simulink model "arduino_encoder"  (R2023b)
settings: Solver=FixedStepAuto  StartTime=0.0  StopTime=inf  RelTol=1e-3  EnableMultiTasking=on
undefined symbols (not defined in the file): DiscIntNeverNeededParam
libraries: arduinosensorlib x2
settings Model: ExtModeTrigDuration=2  Creator=yoany  LastModifiedBy=yoany
settings SolverCC: AutoInsertRateTranBlk=on
settings OptimizationCC: EnhancedBackFolding=on  PassReuseOutputArgsAs=Individual arguments  ZeroExternalMemoryAtStartup=off  ZeroInternalMemoryAtStartup=off  MaxStackSize=64  OptimizeBlockOrder=speed  DifferentSizesBufferReuse=on  OptimizationCustomize=off  EfficientTunableParamExpr=on
settings DebuggingCC: ParameterTunabilityLossMsg=error
settings HardwareCC: ProdBitPerPointer=32  ProdBitPerSizeT=32  ProdBitPerPtrDiffT=32  ProdLargestAtomicInteger=Long  ProdLargestAtomicFloat=Double  ProdWordSize=32  ProdHWDeviceType=ARM Compatible->ARM Cortex  UseEmbeddedCoderFeatures=off
settings SFSimCC: MATLABDynamicMemAlloc=off
settings RTWCC: Description=Embedded Coder  SystemTargetFile=ert.tlc  HardwareBoard=Arduino Nano 33 IoT  TemplateMakefile=ert_default_tmf  Toolchain=Arduino ARM  BuildConfiguration=Faster Runs
settings CodeAppCC: ForceParamTrailComments=on  IgnoreCustomStorageClasses=off  OperatorAnnotations=on  SimulinkDataObjDesc=on  SFDataObjDesc=on  InsertBlockDesc=on
settings ERTTargetCC: SupportContinuousTime=on  SupportNonInlinedSFcns=on  SupportVariableSizeSignals=on  ExtModeTransport=3  ExtModeStaticAlloc=on  ExtModeAutomaticAllocSize=off  ExtModeStaticAllocSize=8192  ExtModeMexFile=ext_xcp  ExtModeIntrfLevel=Level2 - Open

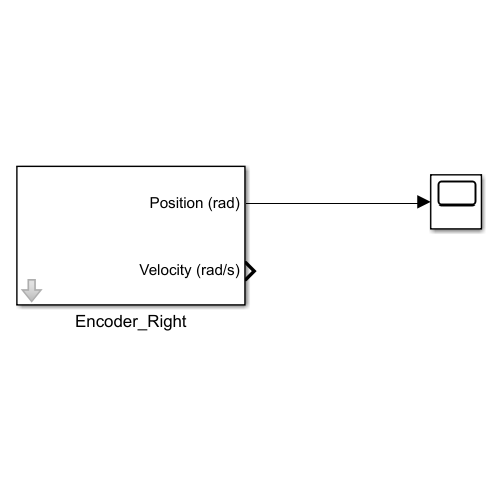
[thumbnail: Simulink's stored preview of the top-level diagram]
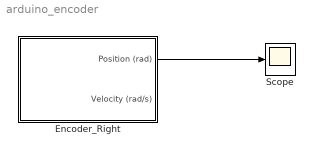
== system arduino_encoder ==
  Encoder_Right : Subsystem  mask{motor_counts_per_rev=67, gear_ratio=90}
      mask prompts: motor_counts_per_rev "Counts Per Rev (in motor)"; gear_ratio "Gear Ratio"
  Scope : Scope
  wires:
  Encoder_Right/1(Position (rad)) -> Scope/1

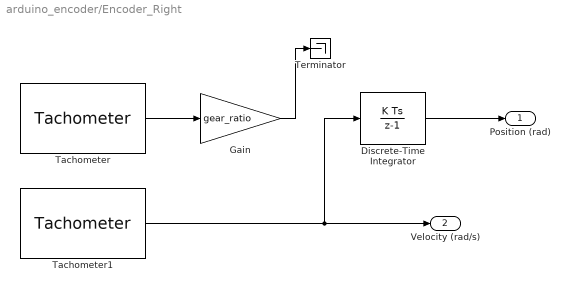
== system arduino_encoder/Encoder_Right ==
  Discrete-Time Integrator : DiscreteIntegrator  SampleTime=0.5  ICPrevOutput=DiscIntNeverNeededParam  ICPrevScaledInput=DiscIntNeverNeededParam
  Gain : Gain  Gain=gear_ratio
  Tachometer : arduinosensorlib/Tachometer  PinNumber=10  InterruptMode=RISING  PulseCountperRotation=motor_counts_per_rev  SampleTime=0.5  blockPlatform=ARDUINO
  Tachometer1 : arduinosensorlib/Tachometer  PinNumber=11  InterruptMode=RISING  PulseCountperRotation=64  SampleTime=0.5  blockPlatform=ARDUINO
  Terminator : Terminator
  Position (rad) : Outport
  Velocity (rad/s) : Outport  Port=2
  wires:
  Tachometer/1 -> Gain/1
  Tachometer1/1 -> Discrete-Time Integrator/1, Velocity (rad/s)/1
  Discrete-Time Integrator/1 -> Position (rad)/1
  Gain/1 -> Terminator/1
